simulink model "delay_test"  (R2013a)
settings: Solver=ode45  StartTime=0.0  StopTime=10.0  RelTol=1e-3
settings Model: Creator=雲棠  LastModifiedBy=雲棠

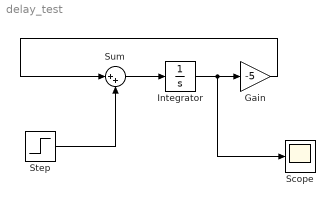
== system delay_test ==
  Gain : Gain  Gain=-5
  Integrator : Integrator  InitialCondition=-2
  Scope : Scope
  Step : Step  SampleTime=0
  Sum : Sum  Inputs=|++
  wires:
  Step/1 -> Sum/2
  Gain/1 -> Sum/1
  Sum/1 -> Integrator/1
  Integrator/1 -> Scope/1, Gain/1
